simulink model "VML_Sim"  (R2019b)
settings: Solver=VariableStepAuto  StartTime=0.0  StopTime=10.0  RelTol=1e-3
libraries: aerolibutil x1, sharedtransform x1
settings Model: Creator=samuelcarbone  LastModifiedBy=samuelcarbone

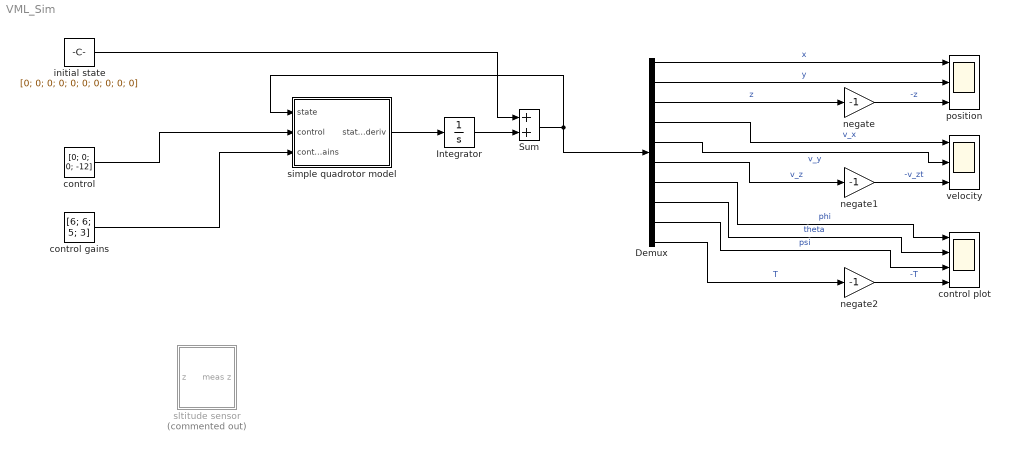
== system VML_Sim ==
  Demux : Demux  Outputs=10
  Integrator : Integrator
  Sum : Sum  Inputs=2
  control : Constant  Value=[0; 0; 0; -12]
  control gains : Constant  Value=[6; 6; 5; 3]
  control plot : Scope  NumInputPorts=4
  initial state : Constant  Value=[0; 0; 0; 0; 0; 0; 0; 0; 0; 0]
  negate : Gain  Gain=-1
  negate1 : Gain  Gain=-1
  negate2 : Gain  Gain=-1
  position : Scope  NumInputPorts=3
  simple quadrotor model : Subsystem
  sltitude sensor : Subsystem  Commented=on
  velocity : Scope  NumInputPorts=3
  wires:
  initial state/1 -> Sum/1
  control/1 -> simple quadrotor model/2(control)
  control gains/1 -> simple quadrotor model/3(control gains)
  simple quadrotor model/1(state deriv) -> Integrator/1
  Integrator/1 -> Sum/2
  Sum/1 -> Demux/1, simple quadrotor model/1(state)
  Demux/10 -> negate2/1  "T"
  Demux/3 -> negate/1  "z"
  Demux/6 -> negate1/1  "v_z"
  negate/1 -> position/3  "-z"
  negate1/1 -> velocity/3  "-v_zt"
  negate2/1 -> control plot/4  "-T"
  Demux/1 -> position/1  "x"
  Demux/2 -> position/2  "y"
  Demux/4 -> velocity/1  "v_x"
  Demux/5 -> velocity/2  "v_y"
  Demux/9 -> control plot/3  "psi"
  Demux/7 -> control plot/1  "phi"
  Demux/8 -> control plot/2  "theta"

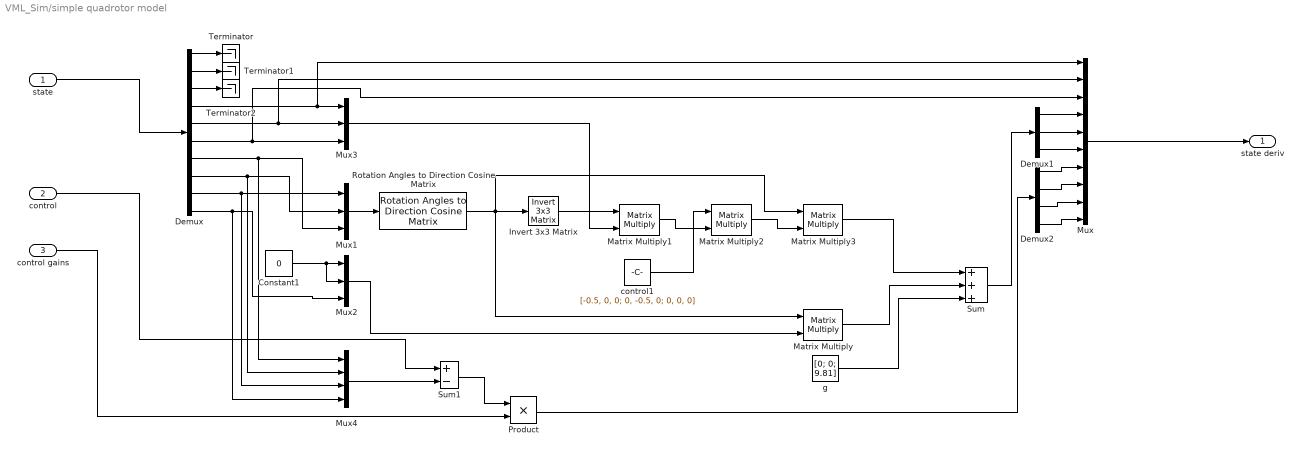
== system VML_Sim/simple quadrotor model ==
  state : Inport
  control : Inport  Port=2
  control gains : Inport  Port=3
  Constant1 : Constant  Value=0
  Demux : Demux  Outputs=10
  Demux1 : Demux  Outputs=3
  Demux2 : Demux
  Invert 3x3 Matrix : aerolibutil/Invert  3x3 Matrix
  Matrix Multiply{,1..3} (4 alike) : Product  Multiplication=Matrix(*)
  Mux : Mux  Inputs=10
  Mux1 : Mux  Inputs=3
  Mux2 : Mux  Inputs=3
  Mux3 : Mux  Inputs=3
  Mux4 : Mux
  Product : Product
  Rotation Angles to Direction Cosine Matrix : sharedtransform/Rotation Angles to Direction Cosine Matrix  rotationOrder=ZYX  aMode=aMode
      settings: SourceProductBaseCode=AE
  Sum : Sum  Inputs=+++
  Sum1 : Sum  Inputs=+-
  Terminator : Terminator
  Terminator1 : Terminator
  Terminator2 : Terminator
  control1 : Constant  Value=[-0.5, 0, 0; 0, -0.5, 0; 0, 0, 0]
  g : Constant  Value=[0; 0; 9.81]
  state deriv : Outport
  wires:
  control gains/1 -> Product/2
  Demux/3 -> Terminator2/1
  Product/1 -> Demux2/1
  Mux1/1 -> Rotation Angles to Direction Cosine Matrix/1
  Mux2/1 -> Matrix Multiply/2
  control/1 -> Sum1/1
  Demux2/1 -> Mux/7
  Constant1/1 -> Mux2/2, Mux2/1
  Matrix Multiply/1 -> Sum/2
  Mux4/1 -> Sum1/2
  control1/1 -> Matrix Multiply2/1
  Matrix Multiply1/1 -> Matrix Multiply2/2
  Sum/1 -> Demux1/1
  state/1 -> Demux/1
  Demux/1 -> Terminator/1
  Demux/9 -> Mux4/3, Mux1/1
  Demux/2 -> Terminator1/1
  Demux/7 -> Mux4/1, Mux1/3
  Matrix Multiply3/1 -> Sum/1
  Demux2/3 -> Mux/9
  Demux/4 -> Mux3/1, Mux/1
  Matrix Multiply2/1 -> Matrix Multiply3/2
  Demux1/3 -> Mux/6
  Demux1/1 -> Mux/4
  Demux/6 -> Mux3/3, Mux/3
  Invert 3x3 Matrix/1 -> Matrix Multiply1/1
  Demux2/2 -> Mux/8
  Demux1/2 -> Mux/5
  Demux/10 -> Mux4/4, Mux2/3
  Rotation Angles to Direction Cosine Matrix/1 -> Matrix Multiply/1, Matrix Multiply3/1, Invert 3x3 Matrix/1
  Demux2/4 -> Mux/10
  g/1 -> Sum/3
  Demux/5 -> Mux3/2, Mux/2
  Mux3/1 -> Matrix Multiply1/2
  Sum1/1 -> Product/1
  Mux/1 -> state deriv/1
  Demux/8 -> Mux4/2, Mux1/2

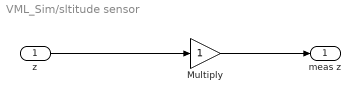
== system VML_Sim/sltitude sensor ==
  z : Inport
  Multiply : Gain
  meas z : Outport
  wires:
  z/1 -> Multiply/1
  Multiply/1 -> meas z/1
